simulink model "DynamicWeightCalculation_TestModel"  (R2014a)
settings: Solver=ode45  StartTime=0.0  StopTime=10  MinStep=0.01  RelTol=1e-3
libraries: rocket_dynamic_data_library x1
settings Model: Creator=scorpii  LastModifiedBy=scorpii
settings SolverCC: InitialStep=0.01

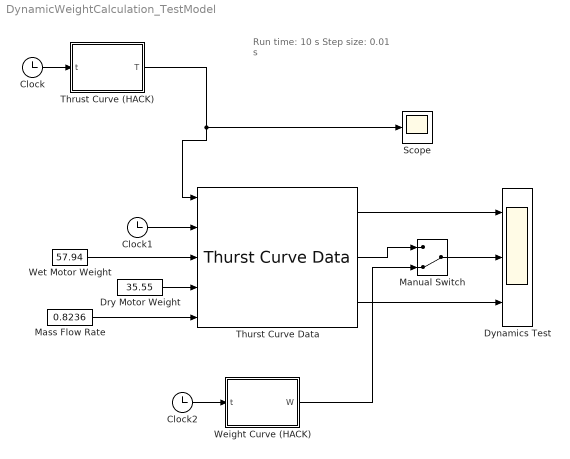
== system DynamicWeightCalculation_TestModel ==
  note: Run time: 10 s
      | Step size: 0.01 s
  Clock : Clock
  Clock1 : Clock
  Clock2 : Clock
  Dry Motor Weight : Constant  Value=35.55
  Dynamics Test : Scope  NumInputPorts=3
      settings: YMin=0~-5~-5  YMax=2400~5~5
  Manual Switch : ManualSwitch  CurrentSetting=0
  Mass Flow Rate : Constant  Value=0.8236
  Scope : Scope
  Thrust Curve (HACK) : MATLAB Function  TreatAsAtomicUnit=on
  Thurst Curve Data : rocket_dynamic_data_library/Thurst Curve Data
  Weight Curve (HACK) : MATLAB Function  TreatAsAtomicUnit=on
  Wet Motor Weight : Constant  Value=57.94
  wires:
  Thurst Curve Data/1 -> Dynamics Test/1
  Thrust Curve (HACK)/1(T) -> Thurst Curve Data/1, Scope/1
  Clock/1 -> Thrust Curve (HACK)/1(t)
  Clock1/1 -> Thurst Curve Data/2
  Dry Motor Weight/1 -> Thurst Curve Data/4
  Wet Motor Weight/1 -> Thurst Curve Data/3
  Mass Flow Rate/1 -> Thurst Curve Data/5
  Thurst Curve Data/3 -> Dynamics Test/3
  Manual Switch/1 -> Dynamics Test/2
  Thurst Curve Data/2 -> Manual Switch/1
  Weight Curve (HACK)/1(W) -> Manual Switch/2
  Clock2/1 -> Weight Curve (HACK)/1(t)

== matlab function DynamicWeightCalculation_TestModel/Weight Curve (HACK) ==
  data: W output; t input
function W = weight_hack(t)

if t<0.47775
    W=(-36625*t^4+32622*t^3-9361.4*t^2-112.87*t+21203)/1000*9.80665 
elseif t<4.0777
    W=(60.388*t^2-1213.3*t+21312)/1000*9.80665 
elseif t<4.5777
    W=(-144.73*t+18078)/1000*9.80665 
else
    W=17422/1000*9.80665 
end

end

== matlab function DynamicWeightCalculation_TestModel/Thrust Curve (HACK) ==
  data: t input; T output
function T = thrust_hack(t)
    if t<0.08
    T=4000000*t^3-462933*t^2+41915*t+209.66
    elseif t<0.15935
    T=-4701*t+2748.7
    elseif t<0.21276 
    T=-1133.2*t+2223.6 
    elseif t<0.32775
    T=787.15*t+1850.2
    elseif t<0.57775
    T=-754.4*t+2339.9
    elseif t<0.72775
    T=-251*t+2070.7 
    elseif t<1.7277
    T=-70.147*t+1947.4
    elseif t<3.3777
    T=-31.421*t^2-9.1503*t+1930.8
    elseif t<3.9777
    T=3656.6*t^3-39167*t^2+137806*t-158018
    elseif t<4.5277
    T=-1051.8*t+4709.4
    else
    T=0
end
